simulink model "Model2D"  (R2024b)
settings: Solver=VariableStepAuto  StartTime=0.0  StopTime=10.0  RelTol=1e-3
undefined symbols (not defined in the file or in its folder): AC, Aero, mot, prop, rad, s, Vbi
libraries: aerolibasang x3, aerolibconvert2 x3, aerolibactuator x3, aerolibtransform2 x2, shared6dof x1, aerolibadyn x1, vrlib x1
settings Model: Creator=Tyler  LastModifiedBy=Tyler

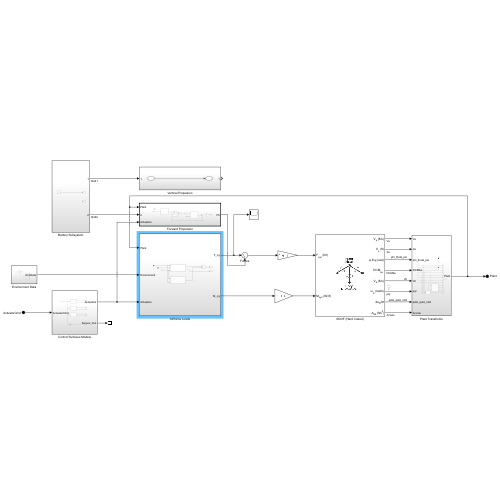
[thumbnail: Simulink's stored preview of the top-level diagram]
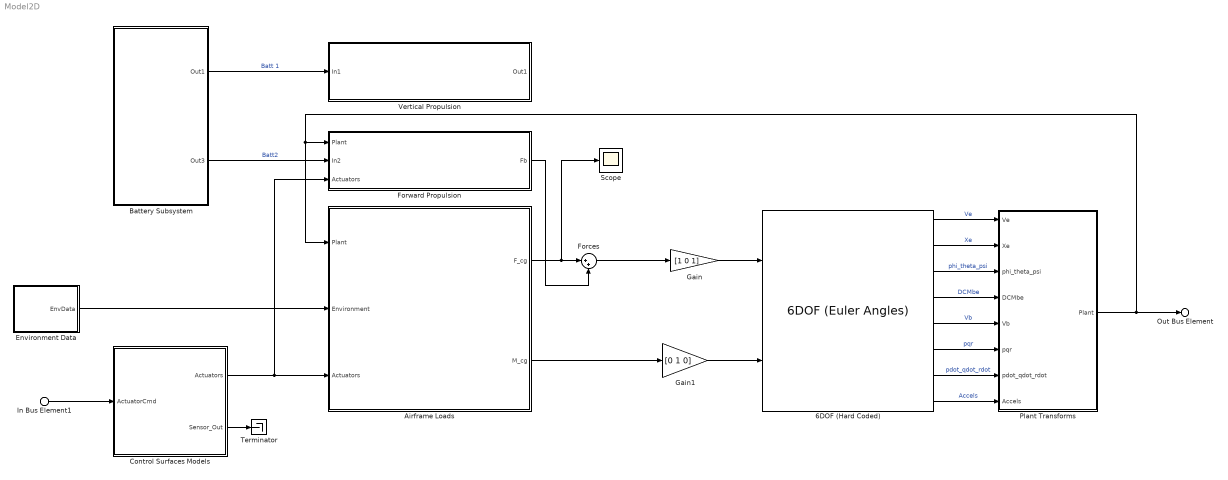
== system Model2D ==
  In Bus Element1 : Inport  PortName=ActuatorCmd
  6DOF (Hard Coded) : shared6dof/6DOF (Euler Angles)  units=English (Velocity in ft/s)  mtype=Fixed  rep=Quaternion  xme_0=[0 0 0]  Vm_0=[0 0 0]  eul_0=[0 0 0]  pm_0=[0 0 0]  mass_0=0.115  mass_e=0.5  mass_f=2.0  inertia=diag([11.38 9.6 20.40])  inertia_e=eye(3)  inertia_f=2*eye(3)  k_quat=1.0  vre_flag=on  abi_flag=off  aMode=0  xme_statename=''  Vm_statename=''  eul_statename=''  quat_statename=''  pm_statename=''  mass_statename=''
  Airframe Loads : Subsystem
  Battery Subsystem : Subsystem
  Control Surfaces Models : Subsystem
  Environment Data : Subsystem
  Forces : Sum  Inputs=|++
  Forward Propulsion : Subsystem  TreatAsAtomicUnit=on
  Gain : Gain  Gain=[1 0 1]
  Gain1 : Gain  Gain=[0 1 0]
  Plant Transforms : Subsystem
  Scope : Scope
  Terminator : Terminator
  Vertical Propulsion : Subsystem
  Out Bus Element : Outport  PortName=Plant
  wires:
  Control Surfaces Models/1(Actuators) -> Airframe Loads/3(Actuators), Forward Propulsion/3(Actuators)
  6DOF (Hard Coded)/6 -> Plant Transforms/6(pqr)  "pqr"
  6DOF (Hard Coded)/3 -> Plant Transforms/3(phi_theta_psi)  "phi_theta_psi"
  6DOF (Hard Coded)/1 -> Plant Transforms/1(Ve)  "Ve"
  Battery Subsystem/2(Out3) -> Forward Propulsion/2(In2)  "Batt2"
  Plant Transforms/1(Plant) -> Out Bus Element/1, Airframe Loads/1(Plant), Forward Propulsion/1(Plant)
  Forward Propulsion/1(Fb) -> Forces/2
  6DOF (Hard Coded)/8 -> Plant Transforms/8(Accels)  "Accels"
  6DOF (Hard Coded)/7 -> Plant Transforms/7(pdot_qdot_rdot)  "pdot_qdot_rdot"
  Gain/1 -> 6DOF (Hard Coded)/1
  6DOF (Hard Coded)/5 -> Plant Transforms/5(Vb)  "Vb"
  Forces/1 -> Gain/1
  Environment Data/1(EnvData) -> Airframe Loads/2(Environment)
  Gain1/1 -> 6DOF (Hard Coded)/2
  6DOF (Hard Coded)/4 -> Plant Transforms/4(DCMbe)  "DCMbe"
  Airframe Loads/2(M_cg) -> Gain1/1
  Control Surfaces Models/2(Sensor_Out) -> Terminator/1
  6DOF (Hard Coded)/2 -> Plant Transforms/2(Xe)  "Xe"
  In Bus Element1/1 -> Control Surfaces Models/1(ActuatorCmd)
  Battery Subsystem/1(Out1) -> Vertical Propulsion/1(In1)  "Batt 1"
  Airframe Loads/1(F_cg) -> Scope/1, Forces/1

== system Model2D/Airframe Loads ==
  Plant : Inport
  In Bus Element : Inport  Port=2  PortName=Environment
  In Bus Element1 : Inport  Port=3  PortName=Actuators
  Add : Sum
  Aerodynamic Loads : Subsystem
  Gravity Force : Subsystem
  F_cg : Outport
  M_cg : Outport  Port=2
  wires:
  Plant/1 -> Gravity Force/1(Plant), Aerodynamic Loads/3(plant)
  In Bus Element/1 -> Gravity Force/2(Environment), Aerodynamic Loads/1(EnvData)
  In Bus Element1/1 -> Aerodynamic Loads/2(Actuators)
  Aerodynamic Loads/1(Fb) -> Add/1
  Add/1 -> F_cg/1
  Aerodynamic Loads/2(Mb) -> M_cg/1
  Gravity Force/1(Fg_b) -> Add/2

== system Model2D/Battery Subsystem ==
  Initial Voltage : Constant
  Out1 : Outport
  Out3 : Outport  Port=2
  wires:
  Initial Voltage/1 -> Out1/1

== system Model2D/Control Surfaces Models ==
  In Bus Element1 : Inport  PortName=ActuatorCmd
  Ailerons : Subsystem
  Bus Selector : BusSelector  OutputSignals=Throttle
  Elevator : Subsystem
  Rudder : Subsystem
  Out Bus Element2 : Outport  VectorParamsAs1DForOutWhenUnconnected=off  PortName=Actuators  Element=Aileron
  Out Bus Element3 : Outport  VectorParamsAs1DForOutWhenUnconnected=off  PortName=Actuators  Element=Elevator
  Out Bus Element4 : Outport  VectorParamsAs1DForOutWhenUnconnected=off  PortName=Actuators  Element=Rudder
  BusElementOut : Outport  PortName=Actuators  Element=Throttle
  Out Bus Element12 : Outport  Port=2  VectorParamsAs1DForOutWhenUnconnected=off  PortName=Sensor_Out  Element=Ail
  Out Bus Element1 : Outport  Port=2  VectorParamsAs1DForOutWhenUnconnected=off  PortName=Sensor_Out  Element=Ele
  Out Bus Element5 : Outport  Port=2  VectorParamsAs1DForOutWhenUnconnected=off  PortName=Sensor_Out  Element=Rud
  wires:
  Ailerons/1(SensorOut) -> Out Bus Element12/1  "Rudder"
  Ailerons/2(Positions) -> Out Bus Element2/1  "Rudder"
  In Bus Element1/1 -> Bus Selector/1, Rudder/1(Commands), Elevator/1(Commands), Ailerons/1(Commands)
  Elevator/1(SensorOut) -> Out Bus Element1/1  "Rudder"
  Elevator/2(Positions) -> Out Bus Element3/1  "Rudder"
  Rudder/2(Positions) -> Out Bus Element4/1  "Rudder"
  Rudder/1(SensorOut) -> Out Bus Element5/1  "Rudder"
  Bus Selector/1 -> BusElementOut/1  "<Throttle>"

== system Model2D/Environment Data ==
  Air Density : Constant  Value=0.002377
  Bus Creator : BusCreator  Inputs=5
  Constant : Constant  Value=0
  Constant1 : Constant  Value=0
  Constant2 : Constant  Value=32.2
  Gravity Acceleration : Constant  Value=[0 0 32.2]
  Mux : Mux  Inputs=3
  Speed of Sound : Constant  Value=1100
  Wind Angular Rates : Constant  Value=[0 0 0]
  Wind Velocity : Constant  Value=[0 0 0]
  EnvData : Outport
  wires:
  Air Density/1 -> Bus Creator/3  "rho"
  Speed of Sound/1 -> Bus Creator/2  "a"
  Mux/1 -> Bus Creator/1  "Ag"
  Wind Velocity/1 -> Bus Creator/4  "WindVelocity"
  Wind Angular Rates/1 -> Bus Creator/5  "WindAngularRates"
  Bus Creator/1 -> EnvData/1  "Environment"
  Constant/1 -> Mux/1
  Constant1/1 -> Mux/2
  Constant2/1 -> Mux/3

== system Model2D/Forward Propulsion ==
  In Bus Element2 : Inport  PortName=Plant  Element=Airspeed
  In2 : Inport  Port=2
  In Bus Element1 : Inport  Port=3  PortName=Actuators  Element=Throttle
  Bus Selector1 : BusSelector  OutputSignals=Thrust,Torque
  Divide1 : Product  Inputs=*/
  Gain1 : Gain  Gain=[1 0 0]
  Integrator : Integrator  InitialCondition=200
  Motor Model : Subsystem
  Prop MOI (slug-ft^2) : Constant  Value=prop.MOI
  Propeller Model : Subsystem
  Subtract : Sum  Inputs=+-
  Fb : Outport
  wires:
  In Bus Element2/1 -> Propeller Model/2(Airspeed)
  Propeller Model/1(Propulsion Data) -> Bus Selector1/1
  Prop MOI (slug-ft^2)/1 -> Divide1/2
  Divide1/1 -> Integrator/1  "Omega dot"
  In Bus Element1/1 -> Motor Model/1(Throttle)
  Integrator/1 -> Propeller Model/1(Omega)  "omega"
  Subtract/1 -> Divide1/1
  Motor Model/1(Torque (ft-lbf)) -> Subtract/1
  Bus Selector1/2 -> Subtract/2  "<Torque>"
  Bus Selector1/1 -> Gain1/1  "<Thrust>"
  Gain1/1 -> Fb/1

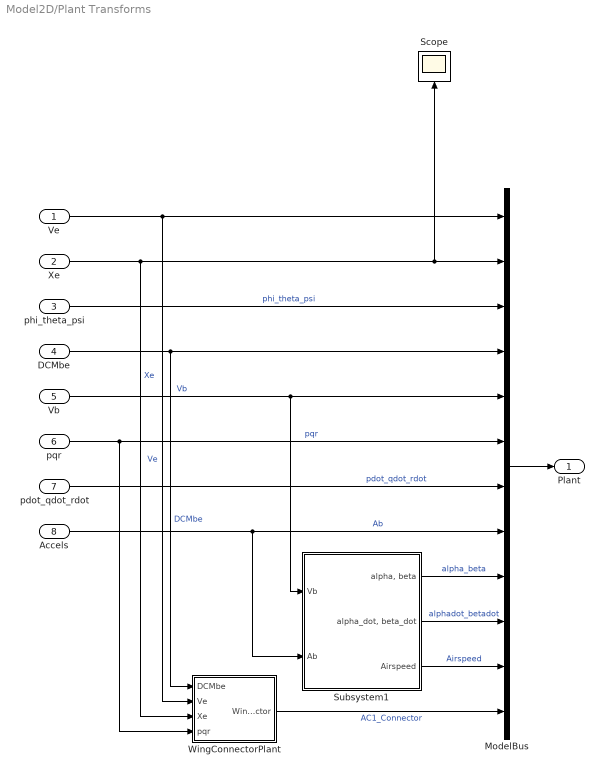
== system Model2D/Plant Transforms ==
  Ve : Inport
  Xe : Inport  Port=2
  phi_theta_psi : Inport  Port=3
  DCMbe : Inport  Port=4
  Vb : Inport  Port=5
  pqr : Inport  Port=6
  pdot_qdot_rdot : Inport  Port=7
  Accels : Inport  Port=8
  ModelBus : BusCreator  Inputs=12
  Scope : Scope
  Subsystem1 : Subsystem
  WingConnectorPlant : Subsystem
  Plant : Outport
  wires:
  Ve/1 -> WingConnectorPlant/2(Ve), ModelBus/1  "Ve"
  ModelBus/1 -> Plant/1
  DCMbe/1 -> ModelBus/4, WingConnectorPlant/1(DCMbe)  "DCMbe"
  pqr/1 -> WingConnectorPlant/4(pqr), ModelBus/6  "pqr"
  pdot_qdot_rdot/1 -> ModelBus/7  "pdot_qdot_rdot"
  Subsystem1/2("alpha_dot, beta_dot") -> ModelBus/10  "alphadot_betadot"
  WingConnectorPlant/1(WingConnector) -> ModelBus/12  "AC1_Connector"
  Xe/1 -> WingConnectorPlant/3(Xe), ModelBus/2, Scope/1  "Xe"
  Subsystem1/1("alpha, beta") -> ModelBus/9  "alpha_beta"
  phi_theta_psi/1 -> ModelBus/3  "phi_theta_psi"
  Accels/1 -> Subsystem1/2(Ab), ModelBus/8  "Ab"
  Vb/1 -> Subsystem1/1(Vb), ModelBus/5  "Vb"
  Subsystem1/3(Airspeed) -> ModelBus/11  "Airspeed"

== system Model2D/Vertical Propulsion ==
  In1 : Inport
  Out1 : Outport
  wires:
  In1/1 -> Out1/1

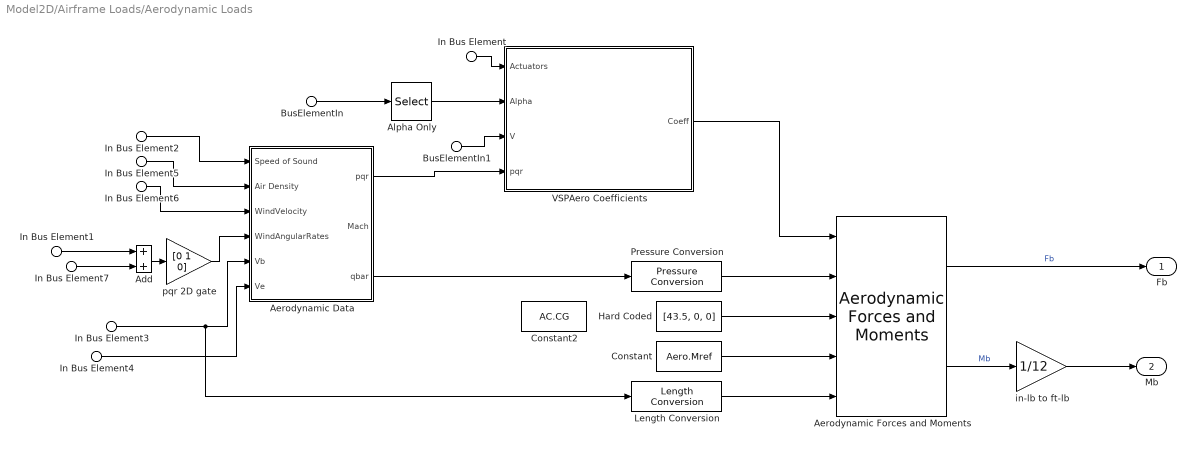
== system Model2D/Airframe Loads/Aerodynamic Loads ==
  In Bus Element6 : Inport  PortName=EnvData  Element=WindVelocity
  In Bus Element7 : Inport  PortName=EnvData  Element=WindAngularRates
  In Bus Element2 : Inport  PortName=EnvData  Element=a
  In Bus Element5 : Inport  PortName=EnvData  Element=rho
  In Bus Element : Inport  Port=2  PortName=Actuators
  In Bus Element3 : Inport  Port=3  PortName=plant  Element=Vb
  In Bus Element4 : Inport  Port=3  PortName=plant  Element=Ve
  In Bus Element1 : Inport  Port=3  PortName=plant  Element=pqr
  BusElementIn : Inport  Port=3  PortName=plant  Element=alpha_beta
  BusElementIn1 : Inport  Port=3  PortName=plant  Element=Airspeed
  Add : Sum
  Aerodynamic Forces and Moments : aerolibadyn/Aerodynamic Forces and Moments   inputAxes=Wind  outputForceAxes=Body  outputMomentAxes=Body  S=Aero.Sref  b=Aero.bref  cbar=Aero.Cref
  Aerodynamic Data : Subsystem
  Alpha Only : Selector  InputPortWidth=2  IndexOptions=Index vector (dialog)  Indices=[1]  OutputSizes=1
  Constant : Constant  Value=Aero.Mref
  Constant2 : Constant  Value=AC.CG
  Hard Coded : Constant  Value=[43.5, 0, 0]
  Length Conversion : aerolibconvert2/Length Conversion  IU=ft  OU=in
  Pressure Conversion : aerolibconvert2/Pressure Conversion  IU=psf  OU=psi
  VSPAero Coefficients : Subsystem
  in-lb to ft-lb : Gain  Gain=1/12
  pqr 2D gate : Gain  Gain=[0 1 0]
  Fb : Outport  VectorParamsAs1DForOutWhenUnconnected=off
  Mb : Outport  Port=2  VectorParamsAs1DForOutWhenUnconnected=off
  wires:
  In Bus Element6/1 -> Aerodynamic Data/3(WindVelocity)
  Aerodynamic Data/1("pqr ") -> VSPAero Coefficients/4(pqr)
  Aerodynamic Forces and Moments/2 -> in-lb to ft-lb/1  "Mb"
  VSPAero Coefficients/1(Coeff) -> Aerodynamic Forces and Moments/1
  In Bus Element7/1 -> Add/2
  Constant/1 -> Aerodynamic Forces and Moments/4
  In Bus Element5/1 -> Aerodynamic Data/2(Air Density)
  In Bus Element2/1 -> Aerodynamic Data/1(Speed of Sound)
  In Bus Element4/1 -> Aerodynamic Data/6(Ve)
  Aerodynamic Forces and Moments/1 -> Fb/1  "Fb"
  In Bus Element1/1 -> Add/1
  In Bus Element/1 -> VSPAero Coefficients/1(Actuators)
  BusElementIn1/1 -> VSPAero Coefficients/3(V)
  In Bus Element3/1 -> Aerodynamic Data/5(Vb), Length Conversion/1
  Aerodynamic Data/3(qbar) -> Pressure Conversion/1
  Hard Coded/1 -> Aerodynamic Forces and Moments/3
  Pressure Conversion/1 -> Aerodynamic Forces and Moments/2
  Length Conversion/1 -> Aerodynamic Forces and Moments/5
  in-lb to ft-lb/1 -> Mb/1
  BusElementIn/1 -> Alpha Only/1
  Alpha Only/1 -> VSPAero Coefficients/2(Alpha)
  pqr 2D gate/1 -> Aerodynamic Data/4(WindAngularRates)
  Add/1 -> pqr 2D gate/1

== system Model2D/Airframe Loads/Gravity Force ==
  Plant : Inport
  Bus Element In2 : Inport  Port=2  PortName=Environment
  Acc to Force : Gain  Gain=AC.mass  OutDataTypeStr=Inherit: Same as input  ParamDataTypeStr=Inherit: Same as input
  Bus Selector : BusSelector  OutputSignals=DCMbe
  Bus Selector1 : BusSelector  OutputSignals=Ag
  Constant : Constant  Value=[0 0 32.2]
  Fg_body : Product  Multiplication=Matrix(*)
  Fg_b : Outport
  wires:
  Bus Selector/1 -> Fg_body/1  "<DCMbe>"
  Acc to Force/1 -> Fg_body/2
  Plant/1 -> Bus Selector/1
  Bus Element In2/1 -> Bus Selector1/1
  Bus Selector1/1 -> ?  "<Ag>"
  Fg_body/1 -> Fg_b/1
  Constant/1 -> Acc to Force/1

== system Model2D/Control Surfaces Models/Ailerons ==
  In Bus Element4 : Inport  PortName=Commands  Element=Aileron
  Nonlinear Second-Order Actuator1 : aerolibactuator/Nonlinear Second-Order Actuator  wn_fin=10  z_fin=1  fin_max=20*pi/180  fin_min=-20*pi/180  fin_maxrate=90*pi/180  fin_act_0=0  fin_act_vel=0
  Scope : Scope  NumInputPorts=2
  SensorOut : Outport  VectorParamsAs1DForOutWhenUnconnected=off
  Positions : Outport  Port=2  VectorParamsAs1DForOutWhenUnconnected=off
  wires:
  Nonlinear Second-Order Actuator1/1 -> Positions/1, Scope/2, SensorOut/1
  In Bus Element4/1 -> Scope/1, Nonlinear Second-Order Actuator1/1  "Ail"

== system Model2D/Control Surfaces Models/Elevator ==
  In Bus Element4 : Inport  PortName=Commands  Element=Elevator
  Nonlinear Second-Order Actuator1 : aerolibactuator/Nonlinear Second-Order Actuator  wn_fin=10  z_fin=1  fin_max=20*pi/180  fin_min=-20*pi/180  fin_maxrate=90*pi/180  fin_act_0=0  fin_act_vel=0
  SensorOut : Outport  VectorParamsAs1DForOutWhenUnconnected=off
  Positions : Outport  Port=2  VectorParamsAs1DForOutWhenUnconnected=off
  wires:
  Nonlinear Second-Order Actuator1/1 -> Positions/1, SensorOut/1
  In Bus Element4/1 -> Nonlinear Second-Order Actuator1/1  "Ele"

== system Model2D/Control Surfaces Models/Rudder ==
  In Bus Element4 : Inport  PortName=Commands  Element=Rudder
  Nonlinear Second-Order Actuator1 : aerolibactuator/Nonlinear Second-Order Actuator  wn_fin=10  z_fin=1  fin_max=20*pi/180  fin_min=-20*pi/180  fin_maxrate=90*pi/180  fin_act_0=0  fin_act_vel=0
  SensorOut : Outport  VectorParamsAs1DForOutWhenUnconnected=off
  Positions : Outport  Port=2  VectorParamsAs1DForOutWhenUnconnected=off
  wires:
  Nonlinear Second-Order Actuator1/1 -> Positions/1, SensorOut/1
  In Bus Element4/1 -> Nonlinear Second-Order Actuator1/1  "Rud"

== system Model2D/Forward Propulsion/Motor Model ==
  Throttle : Inport
  Divide : Product  Inputs=*/
  Kv (RPM/V) : Constant  Value=mot.Kv
  Max Current : Gain  Gain=mot.amp
  Mot Efficiency : Gain
  Motor Conversion Constant : Gain  Gain=8.3
  SI Conversion : Gain  Gain=.7376
  Torque (ft-lbf) : Outport
  wires:
  Mot Efficiency/1 -> Torque (ft-lbf)/1  "Torque (ft-lbf)"
  Throttle/1 -> Max Current/1
  Kv (RPM/V)/1 -> Divide/2
  Divide/1 -> Motor Conversion Constant/1
  Max Current/1 -> Divide/1
  Motor Conversion Constant/1 -> SI Conversion/1  "Torque (N.m)"
  SI Conversion/1 -> Mot Efficiency/1  "Torque (ft-lbf)"

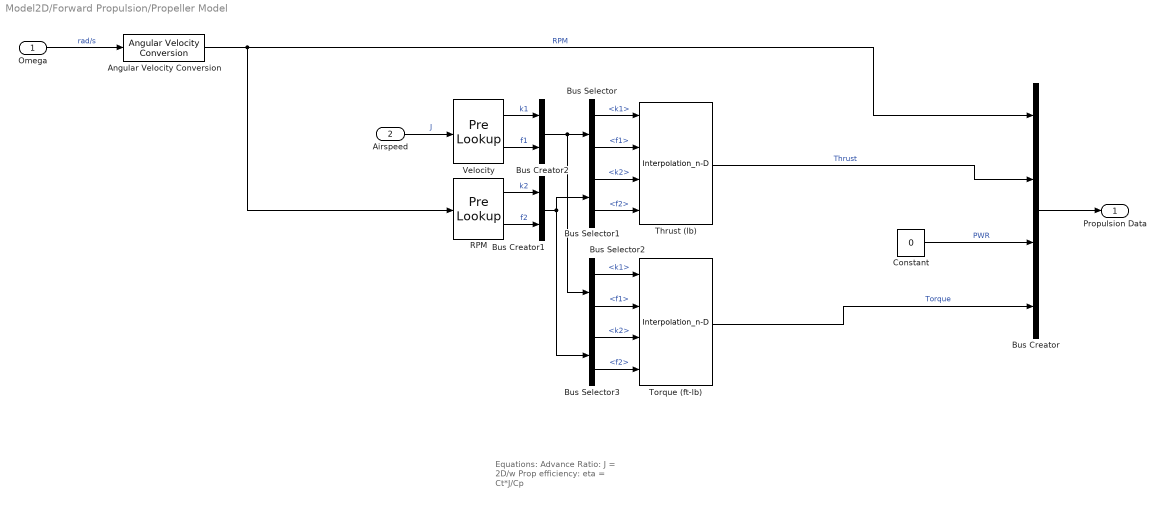
== system Model2D/Forward Propulsion/Propeller Model ==
  note: Equations:
      |
      | Advance Ratio: J = 2D/w
      | Prop efficiency: eta = Ct*J/Cp
  Omega : Inport
  Airspeed : Inport  Port=2
  Angular Velocity Conversion : aerolibconvert2/Angular Velocity Conversion  IU=rad/s  OU=rpm
  Bus Creator : BusCreator  Inputs=4
  Bus Creator1 : BusCreator  Inputs=2
  Bus Creator2 : BusCreator  Inputs=2
  Bus Selector : BusSelector  OutputSignals=k1,f1
  Bus Selector1 : BusSelector  OutputSignals=k2,f2
  Bus Selector2 : BusSelector  OutputSignals=k1,f1
  Bus Selector3 : BusSelector  OutputSignals=k2,f2
  Constant : Constant  Value=0
  RPM : PreLookup  BreakpointsData=prop.RPM  ExtrapMethod=Linear
  Thrust (lb) : Interpolation_n-D  Table=prop.Thrust  InternalRulePriority=Speed
  Torque (ft-lb) : Interpolation_n-D  Table=prop.Torque  ExtrapMethod=Clip  InternalRulePriority=Speed
  Velocity : PreLookup  BreakpointsData=prop.vel
  Propulsion Data : Outport
  wires:
  Constant/1 -> Bus Creator/3  "PWR"
  Torque (ft-lb)/1 -> Bus Creator/4  "Torque"
  Angular Velocity Conversion/1 -> RPM/1, Bus Creator/1  "RPM"
  Bus Creator/1 -> Propulsion Data/1
  Omega/1 -> Angular Velocity Conversion/1  "rad/s"
  Airspeed/1 -> Velocity/1  "J"
  Velocity/2 -> Bus Creator2/2  "f1"
  Bus Creator2/1 -> Bus Selector/1, Bus Selector2/1
  Bus Creator1/1 -> Bus Selector1/1, Bus Selector3/1
  Velocity/1 -> Bus Creator2/1  "k1"
  Bus Selector2/2 -> Torque (ft-lb)/2  "<f1>"
  RPM/1 -> Bus Creator1/1  "k2"
  Bus Selector2/1 -> Torque (ft-lb)/1  "<k1>"
  RPM/2 -> Bus Creator1/2  "f2"
  Thrust (lb)/1 -> Bus Creator/2  "Thrust"
  Bus Selector/2 -> Thrust (lb)/2  "<f1>"
  Bus Selector3/2 -> Torque (ft-lb)/4  "<f2>"
  Bus Selector/1 -> Thrust (lb)/1  "<k1>"
  Bus Selector1/2 -> Thrust (lb)/4  "<f2>"
  Bus Selector3/1 -> Torque (ft-lb)/3  "<k2>"
  Bus Selector1/1 -> Thrust (lb)/3  "<k2>"

== system Model2D/Plant Transforms/Subsystem1 ==
  Vb : Inport
  Ab : Inport  Port=2
  Direction Cosine Matrix Body to Wind : aerolibtransform2/Direction Cosine Matrix Body to Wind
  "Incidence, Sideslip, & Airspeed" : aerolibasang/Incidence, Sideslip, & Airspeed
  Memory4 : Memory  InitialCondition=Vbi
  Mux4 : Mux  Inputs=2
  Product1 : Product  Multiplication=Matrix(*)  InputSameDT=on  SaturateOnIntegerOverflow=on  OutDataTypeStr=Inherit: Same as first input
  "calc alpha_dot, beta_dot" : Subsystem
  "alpha, beta" : Outport  Unit=rad  VectorParamsAs1DForOutWhenUnconnected=off
  "alpha_dot, beta_dot" : Outport  Port=2  Unit=rad/s  VectorParamsAs1DForOutWhenUnconnected=off
  Airspeed : Outport  Port=3
  wires:
  "Incidence, Sideslip, & Airspeed"/2 -> Mux4/2
  Mux4/1 -> "alpha, beta"/1, Direction Cosine Matrix Body to Wind/1, "calc alpha_dot, beta_dot"/1(alpha,beta)
  Direction Cosine Matrix Body to Wind/1 -> Product1/1
  "Incidence, Sideslip, & Airspeed"/1 -> Mux4/1
  Memory4/1 -> Product1/2, "Incidence, Sideslip, & Airspeed"/1
  Product1/1 -> "calc alpha_dot, beta_dot"/3(Vw)
  Ab/1 -> "calc alpha_dot, beta_dot"/2(Ab)
  "Incidence, Sideslip, & Airspeed"/3 -> Airspeed/1
  "calc alpha_dot, beta_dot"/1("alpha_dot, beta_dot") -> "alpha_dot, beta_dot"/1
  Vb/1 -> Memory4/1

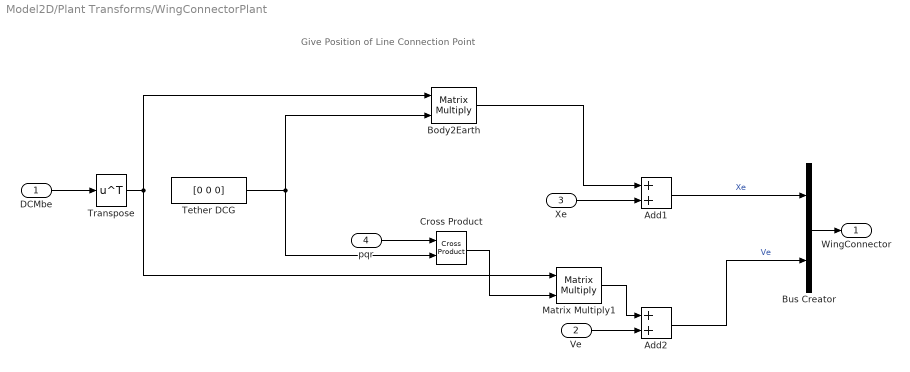
== system Model2D/Plant Transforms/WingConnectorPlant ==
  note: Give Position of Line Connection Point
  DCMbe : Inport
  Ve : Inport  Port=2
  Xe : Inport  Port=3
  pqr : Inport  Port=4
  Add1 : Sum
  Add2 : Sum
  Body2Earth : Product  Multiplication=Matrix(*)
  Bus Creator : BusCreator  Inputs=2
  Cross Product : vrlib/Utilities/Cross Product
  Matrix Multiply1 : Product  Multiplication=Matrix(*)
  Tether DCG : Constant  Value=[0 0 0]
  Transpose : Math  Operator=transpose
  WingConnector : Outport
  wires:
  Bus Creator/1 -> WingConnector/1
  Transpose/1 -> Body2Earth/1, Matrix Multiply1/1
  Body2Earth/1 -> Add1/1
  Add2/1 -> Bus Creator/2  "Ve"
  Xe/1 -> Add1/2
  Matrix Multiply1/1 -> Add2/1
  Tether DCG/1 -> Cross Product/2, Body2Earth/2
  pqr/1 -> Cross Product/1
  Cross Product/1 -> Matrix Multiply1/2
  Add1/1 -> Bus Creator/1  "Xe"
  DCMbe/1 -> Transpose/1
  Ve/1 -> Add2/2

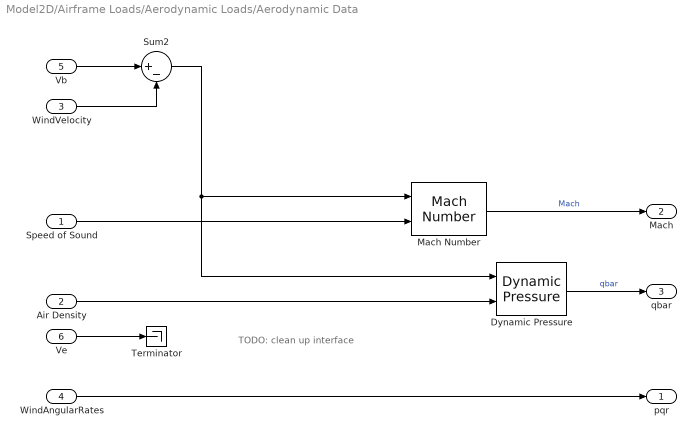
== system Model2D/Airframe Loads/Aerodynamic Loads/Aerodynamic Data ==
  note: TODO: clean up interface
  Speed of Sound : Inport
  Air Density : Inport  Port=2
  WindVelocity : Inport  Port=3  PortDimensions=3
  WindAngularRates : Inport  Port=4  PortDimensions=3
  Vb : Inport  Port=5  PortDimensions=3
  Ve : Inport  Port=6  PortDimensions=3
  Dynamic Pressure : aerolibasang/Dynamic Pressure
  Mach Number : aerolibasang/Mach Number
  Sum2 : Sum  Inputs=|+-  InputSameDT=on  SaturateOnIntegerOverflow=on  OutDataTypeStr=Inherit: Same as first input
  Terminator : Terminator
  "pqr " : Outport  VectorParamsAs1DForOutWhenUnconnected=off
  Mach : Outport  Port=2  VectorParamsAs1DForOutWhenUnconnected=off
  qbar : Outport  Port=3  VectorParamsAs1DForOutWhenUnconnected=off
  wires:
  Dynamic Pressure/1 -> qbar/1  "qbar"
  Sum2/1 -> Mach Number/1, Dynamic Pressure/1
  Ve/1 -> Terminator/1
  Mach Number/1 -> Mach/1  "Mach"
  WindVelocity/1 -> Sum2/2
  Air Density/1 -> Dynamic Pressure/2
  WindAngularRates/1 -> "pqr "/1
  Speed of Sound/1 -> Mach Number/2
  Vb/1 -> Sum2/1

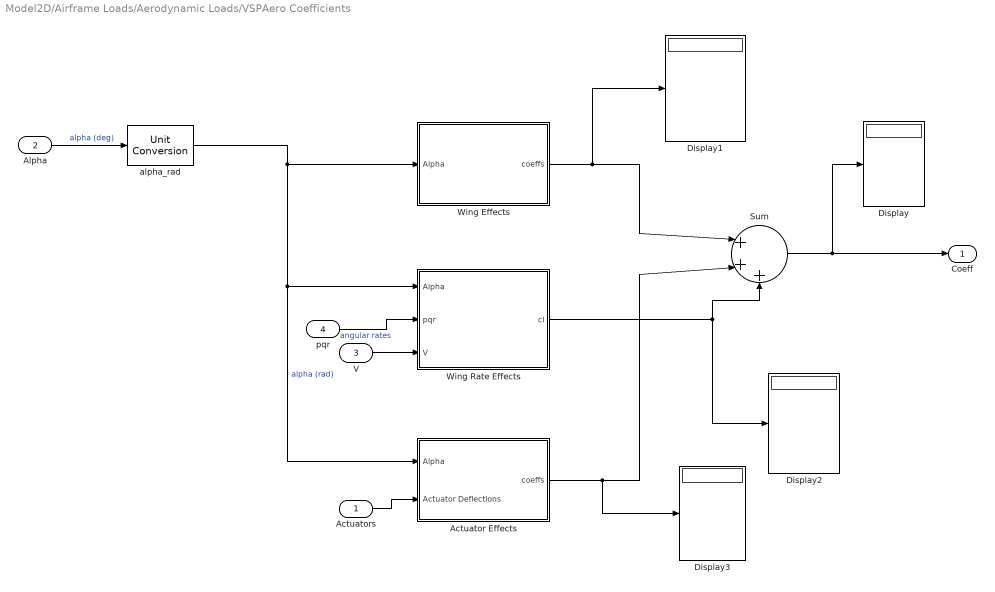
== system Model2D/Airframe Loads/Aerodynamic Loads/VSPAero Coefficients ==
  Actuators : Inport
  Alpha : Inport  Port=2  Unit=rad
  V : Inport  Port=3
  pqr : Inport  Port=4
  Actuator Effects : Subsystem
  Display{,1..3} (4 alike) : Display
  Sum : Sum  Inputs=|+++
  Wing Effects : Subsystem
  Wing Rate Effects : Subsystem
  alpha_rad : UnitConversion
  Coeff : Outport  VectorParamsAs1DForOutWhenUnconnected=off
  wires:
  Wing Rate Effects/1(cl) -> Sum/3, Display2/1
  Sum/1 -> Display/1, Coeff/1
  alpha_rad/1 -> Wing Rate Effects/1(Alpha), Actuator Effects/1(Alpha), Wing Effects/1(Alpha)  "alpha (rad)"
  Actuators/1 -> Actuator Effects/2("Actuator Deflections ")
  V/1 -> Wing Rate Effects/3(V)
  Alpha/1 -> alpha_rad/1  "alpha (deg)"
  Actuator Effects/1(coeffs) -> Sum/2, Display3/1
  pqr/1 -> Wing Rate Effects/2(pqr)  "angular rates"
  Wing Effects/1(coeffs) -> Sum/1, Display1/1

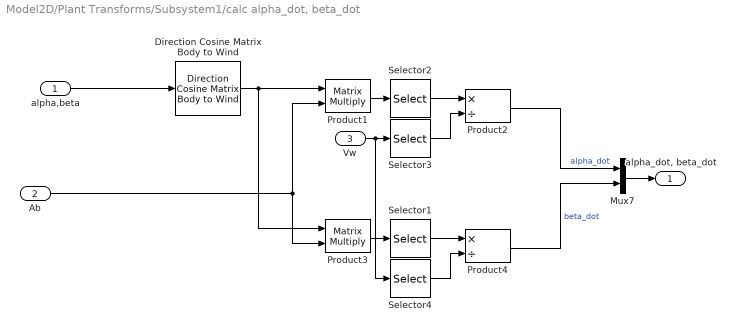
== system Model2D/Plant Transforms/Subsystem1/calc alpha_dot, beta_dot ==
  alpha,beta : Inport
  Ab : Inport  Port=2
  Vw : Inport  Port=3
  Direction Cosine Matrix Body to Wind : aerolibtransform2/Direction Cosine Matrix Body to Wind
  Mux7 : Mux  Inputs=2
  Product1 : Product  Multiplication=Matrix(*)  InputSameDT=on  SaturateOnIntegerOverflow=on  OutDataTypeStr=Inherit: Same as first input
  Product2 : Product  Inputs=*/  InputSameDT=on  SaturateOnIntegerOverflow=on  OutDataTypeStr=Inherit: Same as first input
  Product3 : Product  Multiplication=Matrix(*)  InputSameDT=on  SaturateOnIntegerOverflow=on  OutDataTypeStr=Inherit: Same as first input
  Product4 : Product  Inputs=*/  InputSameDT=on  SaturateOnIntegerOverflow=on  OutDataTypeStr=Inherit: Same as first input
  Selector1 : Selector  IndexMode=Zero-based  InputPortWidth=3  IndexOptions=Index vector (dialog)  Indices=1  OutputSizes=1
  Selector2 : Selector  IndexMode=Zero-based  InputPortWidth=3  IndexOptions=Index vector (dialog)  Indices=2  OutputSizes=1
  Selector3 : Selector  IndexMode=Zero-based  InputPortWidth=3  IndexOptions=Index vector (dialog)  Indices=0  OutputSizes=1
  Selector4 : Selector  IndexMode=Zero-based  InputPortWidth=3  IndexOptions=Index vector (dialog)  Indices=0  OutputSizes=1
  "alpha_dot, beta_dot" : Outport  VectorParamsAs1DForOutWhenUnconnected=off
  wires:
  Product1/1 -> Selector2/1
  Selector2/1 -> Product2/1
  Selector3/1 -> Product2/2
  alpha,beta/1 -> Direction Cosine Matrix Body to Wind/1
  Product2/1 -> Mux7/1  "alpha_dot"
  Ab/1 -> Product1/2, Product3/2
  Vw/1 -> Selector4/1, Selector3/1
  Product4/1 -> Mux7/2  "beta_dot"
  Direction Cosine Matrix Body to Wind/1 -> Product3/1, Product1/1
  Selector1/1 -> Product4/1
  Selector4/1 -> Product4/2
  Product3/1 -> Selector1/1
  Mux7/1 -> "alpha_dot, beta_dot"/1

== system Model2D/Airframe Loads/Aerodynamic Loads/VSPAero Coefficients/Actuator Effects ==
  note: Constant blocks commented out for inputs of finalized model
  Alpha : Inport  Unit=deg
  "Actuator Deflections " : Inport  Port=2
  Add : Sum
  Ailerons : Subsystem
  AlphaLookup : PreLookup  Commented=on  BreakpointsData=Aero.alpha_vec  BeginIndexSearchUsingPreviousIndexResult=on  ExtrapMethod=Linear
  Bus Creator : BusCreator  Commented=on  Inputs=2
  Constant1 : Constant  Commented=on  Value=-30
  Constant3 : Constant  Commented=on  Value=-15
  Display : Display
  Elevator : Subsystem
  coeffs : Outport  VectorParamsAs1DForOutWhenUnconnected=off
  wires:
  Add/1 -> Display/1, coeffs/1
  Ailerons/1(delCoeff) -> Add/2
  AlphaLookup/2 -> Bus Creator/2  "f"
  AlphaLookup/1 -> Bus Creator/1  "k"
  "Actuator Deflections "/1 -> Ailerons/2(Actuators), Elevator/2(Actuators)
  Elevator/1(delCoeff) -> Add/1
  Alpha/1 -> Ailerons/1(Alpha), Elevator/1(Alpha)

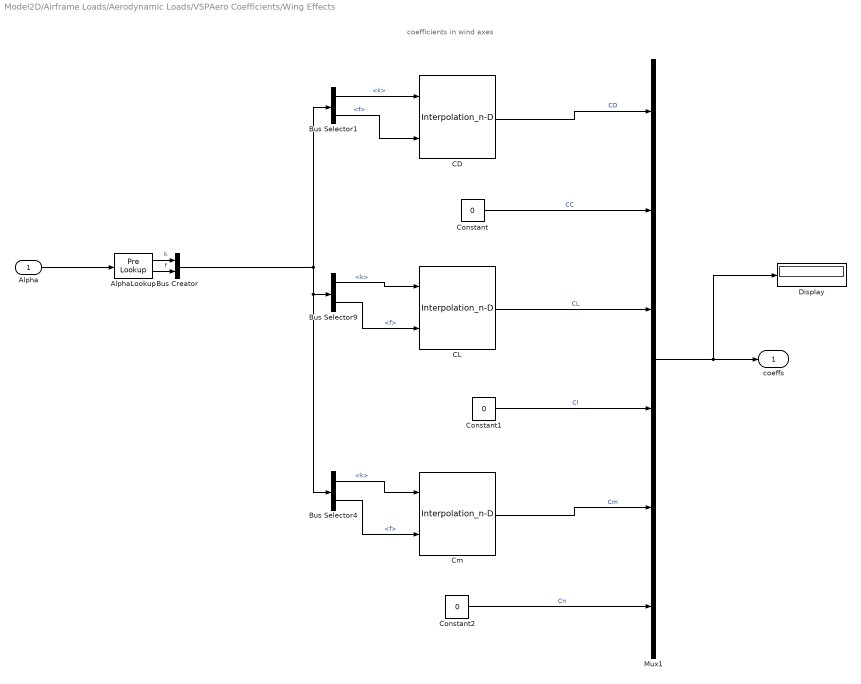
== system Model2D/Airframe Loads/Aerodynamic Loads/VSPAero Coefficients/Wing Effects ==
  note: coefficients in wind axes
  Alpha : Inport  Unit=deg
  AlphaLookup : PreLookup  BreakpointsData=Aero.alpha_vec  BeginIndexSearchUsingPreviousIndexResult=on  ExtrapMethod=Linear
  Bus Creator : BusCreator  Inputs=2
  Bus Selector1 : BusSelector  OutputSignals=k,f
  Bus Selector4 : BusSelector  OutputSignals=k,f
  Bus Selector9 : BusSelector  OutputSignals=k,f
  CD : Interpolation_n-D  NumberOfTableDimensions=1  Table=Aero.CD(find(abs(Aero.beta_vec)==min(abs(Aero.beta_vec)),1),:)  RemoveProtectionIndex=on  SaturateOnIntegerOverflow=on
      settings: InputPortMap=u0,u1
  CL : Interpolation_n-D  NumberOfTableDimensions=1  Table=Aero.CL(find(abs(Aero.beta_vec)==min(abs(Aero.beta_vec)),1),:)  RemoveProtectionIndex=on  SaturateOnIntegerOverflow=on
      settings: InputPortMap=u0,u1
  Cm : Interpolation_n-D  NumberOfTableDimensions=1  Table=Aero.Cm(find(abs(Aero.beta_vec)==min(abs(Aero.beta_vec)),1),:)  RemoveProtectionIndex=on  SaturateOnIntegerOverflow=on
      settings: InputPortMap=u0,u1
  Constant : Constant  Value=0
  Constant1 : Constant  Value=0
  Constant2 : Constant  Value=0
  Display : Display
  Mux1 : Mux  Inputs=6
  coeffs : Outport  VectorParamsAs1DForOutWhenUnconnected=off
  wires:
  AlphaLookup/2 -> Bus Creator/2  "f"
  AlphaLookup/1 -> Bus Creator/1  "k"
  Mux1/1 -> Display/1, coeffs/1
  Alpha/1 -> AlphaLookup/1
  Cm/1 -> Mux1/5  "Cm"
  Bus Selector4/2 -> Cm/2  "<f>"
  Bus Selector1/1 -> CD/1  "<k>"
  CL/1 -> Mux1/3  "CL"
  Bus Selector9/1 -> CL/1  "<k>"
  Bus Selector1/2 -> CD/2  "<f>"
  Constant2/1 -> Mux1/6  "Cn"
  Bus Selector4/1 -> Cm/1  "<k>"
  Bus Creator/1 -> Bus Selector1/1, Bus Selector4/1, Bus Selector9/1
  Constant/1 -> Mux1/2  "CC"
  Bus Selector9/2 -> CL/2  "<f>"
  Constant1/1 -> Mux1/4  "Cl"
  CD/1 -> Mux1/1  "CD"

== system Model2D/Airframe Loads/Aerodynamic Loads/VSPAero Coefficients/Wing Rate Effects ==
  note: Remove these look-up tables when submodels are finalized
  Alpha : Inport  Unit=deg
  pqr : Inport  Port=2
  V : Inport  Port=3
  Aero Surfaces : Subsystem
  AlphaLookup : PreLookup  Commented=on  BreakpointsData=Aero.alpha_vec  BeginIndexSearchUsingPreviousIndexResult=on  ExtrapMethod=Linear
  Bus Creator : BusCreator  Commented=on  Inputs=2
  Display : Display
  Gain : Gain  Gain=Aero.Cref/2
  Product : Product  Inputs=*/
  Scope : Scope
  q only : Selector  InputPortWidth=3  IndexOptions=Index vector (dialog)  Indices=[2]  OutputSizes=1
  cl : Outport  VectorParamsAs1DForOutWhenUnconnected=off
  wires:
  V/1 -> Aero Surfaces/3(V)
  AlphaLookup/2 -> Bus Creator/2  "f"
  AlphaLookup/1 -> Bus Creator/1  "k"
  Aero Surfaces/1(delCoeff) -> Display/1, cl/1, Scope/1
  Alpha/1 -> Aero Surfaces/1(Alpha)
  pqr/1 -> q only/1
  q only/1 -> Gain/1
  Gain/1 -> Product/1

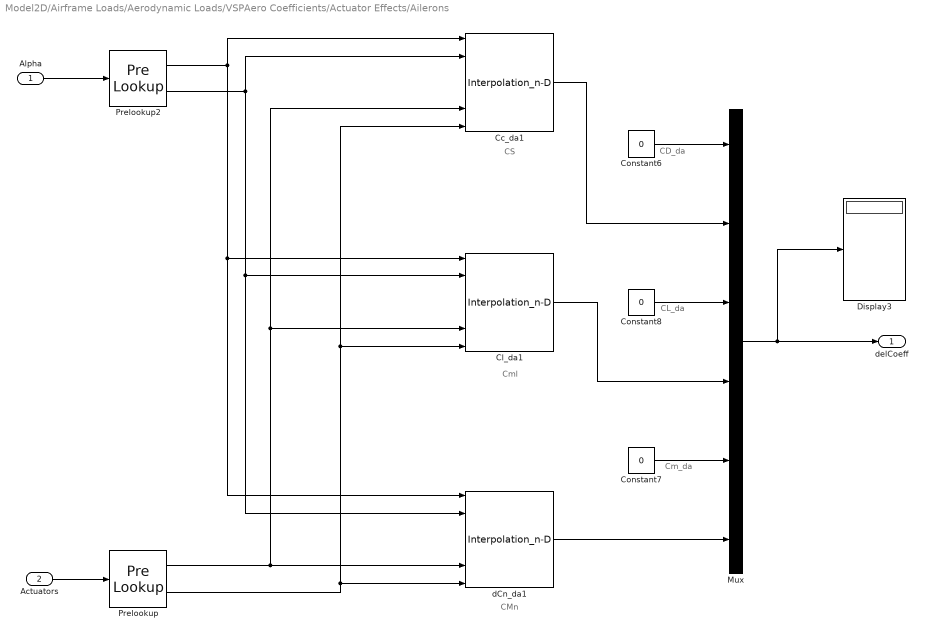
== system Model2D/Airframe Loads/Aerodynamic Loads/VSPAero Coefficients/Actuator Effects/Ailerons ==
  note: CL_da
  note: CD_da
  note: Cm_da
  note: CMn
  note: CS
  note: Cml
  Alpha : Inport
  Actuators : Inport  Port=2
  Cc_da1 : Interpolation_n-D  NumberOfTableDimensions=3  Table=Aero.Cc_da  RemoveProtectionIndex=on  SaturateOnIntegerOverflow=on
      settings: InputPortMap=u0,u1,u2,u3,u4,u5
  Cl_da1 : Interpolation_n-D  NumberOfTableDimensions=3  Table=Aero.Cl_da  RemoveProtectionIndex=on  SaturateOnIntegerOverflow=on
      settings: InputPortMap=u0,u1,u2,u3,u4,u5
  Constant6 : Constant  Value=0
  Constant7 : Constant  Value=0
  Constant8 : Constant  Value=0
  Display3 : Display
  Mux : Mux  Inputs=6
  Prelookup : PreLookup  BreakpointsData=Aero.delta_vec  ExtrapMethod=Linear
  Prelookup2 : PreLookup  BreakpointsData=Aero.alpha_vec  ExtrapMethod=Linear
  dCn_da1 : Interpolation_n-D  NumberOfTableDimensions=3  Table=Aero.Cn_da  RemoveProtectionIndex=on  SaturateOnIntegerOverflow=on
      settings: InputPortMap=u0,u1,u2,u3,u4,u5
  delCoeff : Outport  VectorParamsAs1DForOutWhenUnconnected=off
  wires:
  Constant7/1 -> Mux/5
  Constant6/1 -> Mux/1
  dCn_da1/1 -> Mux/6
  Prelookup2/1 -> dCn_da1/1, Cl_da1/1, Cc_da1/1
  Cc_da1/1 -> Mux/2
  Mux/1 -> delCoeff/1, Display3/1
  Prelookup/1 -> Cc_da1/5, Cl_da1/5, dCn_da1/5
  Prelookup/2 -> Cc_da1/6, Cl_da1/6, dCn_da1/6
  Constant8/1 -> Mux/3
  Prelookup2/2 -> dCn_da1/2, Cl_da1/2, Cc_da1/2
  Cl_da1/1 -> Mux/4
  Actuators/1 -> Prelookup/1
  Alpha/1 -> Prelookup2/1

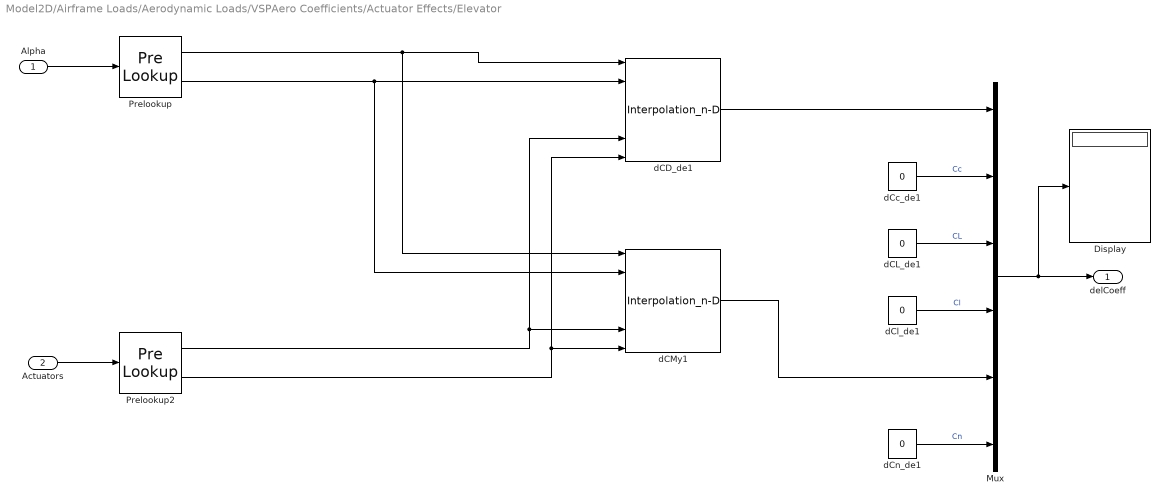
== system Model2D/Airframe Loads/Aerodynamic Loads/VSPAero Coefficients/Actuator Effects/Elevator ==
  Alpha : Inport
  Actuators : Inport  Port=2
  Display : Display
  Mux : Mux  Inputs=6
  Prelookup : PreLookup  BreakpointsData=Aero.alpha_vec  ExtrapMethod=Linear
  Prelookup2 : PreLookup  BreakpointsData=Aero.delta_vec  ExtrapMethod=Linear
  dCD_de1 : Interpolation_n-D  NumberOfTableDimensions=3  Table=Aero.CD_de  RemoveProtectionIndex=on  SaturateOnIntegerOverflow=on
      settings: InputPortMap=u0,u1,u2,u3,u4,u5
  dCL_de1 : Constant  Value=0
  dCMy1 : Interpolation_n-D  NumberOfTableDimensions=3  Table=Aero.Cm_de  RemoveProtectionIndex=on  SaturateOnIntegerOverflow=on
      settings: InputPortMap=u0,u1,u2,u3,u4,u5
  dCc_de1 : Constant  Value=0
  dCl_de1 : Constant  Value=0
  dCn_de1 : Constant  Value=0
  delCoeff : Outport  VectorParamsAs1DForOutWhenUnconnected=off
  wires:
  dCMy1/1 -> Mux/5
  dCn_de1/1 -> Mux/6  "Cn"
  Alpha/1 -> Prelookup/1
  Prelookup2/1 -> dCMy1/5, dCD_de1/5
  Prelookup2/2 -> dCD_de1/6, dCMy1/6
  Prelookup/2 -> dCMy1/2, dCD_de1/2
  dCD_de1/1 -> Mux/1
  dCL_de1/1 -> Mux/3  "CL"
  Prelookup/1 -> dCMy1/1, dCD_de1/1
  dCl_de1/1 -> Mux/4  "Cl"
  Actuators/1 -> Prelookup2/1
  dCc_de1/1 -> Mux/2  "Cc"
  Mux/1 -> delCoeff/1, Display/1

== system Model2D/Airframe Loads/Aerodynamic Loads/VSPAero Coefficients/Wing Rate Effects/Aero Surfaces ==
  note: Display used here to show the Damping Coefficients
      | as a means of ensuring roll, pitch, and yaw rate is correct.
  note: Display for the C_roll, C_pitch, and C_yaw after convert/add.
  Alpha : Inport
  pqr : Inport  Port=2
  V : Inport  Port=3
  Bus Creator : BusCreator  Inputs=3
  "C_roll, C_pitch, C_yaw" : Display
  Coefs Due to Pitch Rate : Subsystem
  Convert & Add : Subsystem
      settings: PortSchema="{\"entries\":[{\"content\":{\"sides\":[{\"content\":{\"connectorIds\":[\"In1\"]},\"type\":\"ConnectorPlacement.EquallySpacedRectSide\",\"uuid\":\"b8013de1-6e73-47c3-a52d-200a37bea422\"},{\"content\":{\"connectorIds\":[\"Out1\"],\"side\":\"RIGHT\"},\"type\":\"ConnectorPlacement.EquallySpacedRectSide\",\"uuid\":\"fcf5ea14-4050-433a-82d6-0b7656ed6099\"},{\"content\":{\"connectorIds\":[\"In2\",\"In3\"],\"side\":\"TOP\"},\"type\":\"ConnectorPlacement.EquallySpacedRectSide\",\"uuid\":\"1c09a769-a85c-46fb-a83d-04bd39ae92ac\"},{\"content\":{\"side\":\"BOTTOM\"},\"type\":\"ConnectorPlacement.EquallySpacedRectSide\",\"uuid\":\"8f4a7c03-2c0e-435b-85d5-b3305cee738f\"}]},\"type\":\"ConnectorPlacement.EquallySpacedConnector\",\"uuid\":\"e7daaf90-0c94-4b5f-ae16-89aa994c358a\"}],\"packageUris\":[\"http://schema.mathworks.com/mf0/Connector/R2020b\"],\"version\":\"1.0\"}"
  Display : Display
  delCoeff : Outport  VectorParamsAs1DForOutWhenUnconnected=off
  wires:
  Bus Creator/1 -> Display/1  "Damp Coef"
  Convert & Add/1(delCoeff) -> "C_roll, C_pitch, C_yaw"/1, delCoeff/1
  Alpha/1 -> Coefs Due to Pitch Rate/1(Alpha)
  V/1 -> Convert & Add/3(V)
  pqr/1 -> Convert & Add/2(pqr)

== system Model2D/Airframe Loads/Aerodynamic Loads/VSPAero Coefficients/Wing Rate Effects/Aero Surfaces/Coefs Due to Pitch Rate ==
  Alpha : Inport
  Cm_q1 : Interpolation_n-D  Table=Aero.Cm_q  ExtrapMethod=Clip  RemoveProtectionIndex=on  SaturateOnIntegerOverflow=on
  Constant{5..9} (5 alike) : Constant  Value=0
  Display : Display
  Gain1 : Gain  Commented=through  Gain=0.1
  Mux2 : Mux  Inputs=6
  Prelookup : PreLookup  BreakpointsData=Aero.alpha_vec  ExtrapMethod=Linear
  Out1 : Outport
  wires:
  Alpha/1 -> Prelookup/1
  Cm_q1/1 -> Gain1/1  "CMy"
  Constant5/1 -> Mux2/2  "Cc_q"
  Constant6/1 -> Mux2/4  "Cl_q"
  Constant7/1 -> Mux2/6  "Cn_q"
  Gain1/1 -> Mux2/5  "Cm_q"
  Mux2/1 -> Out1/1, Display/1
  Prelookup/1 -> Cm_q1/3
  Prelookup/2 -> Cm_q1/4
  Constant8/1 -> Mux2/1  "CD_q"
  Constant9/1 -> Mux2/3  "CL_q"

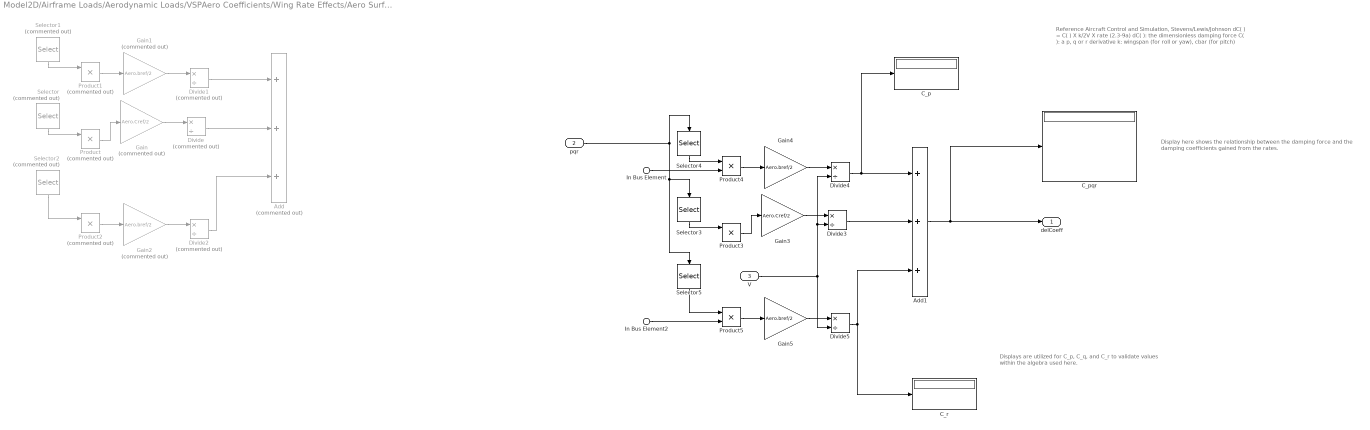
== system Model2D/Airframe Loads/Aerodynamic Loads/VSPAero Coefficients/Wing Rate Effects/Aero Surfaces/Convert & Add ==
  note: Displays are utilized for C_p, C_q, and C_r to validate values
      | within the algebra used here.
  note: Display here shows the relationship between the damping force and
      | the damping coefficients gained from the rates.
  note: Reference Aircraft Control and Simulation, Stevens/Lewis/Johnson
      | dC( ) = C( ) X k/2V X rate    (2.3-9a)
      |
      | dC( ): the dimensionless damping force
      | C( ): a p, q or r derivative
      | k: wingspan (for roll or yaw), cbar (for pitch)
  In Bus Element : Inport  PortName=DampCoef  Element=C()_p
  In Bus Element2 : Inport  PortName=DampCoef  Element=C()_r
  pqr : Inport  Port=2
  V : Inport  Port=3
  Add : Sum  Commented=on  Inputs=+++
  Add1 : Sum  Inputs=+++
  C_p : Display
  C_pqr : Display
  C_r : Display
  Divide : Product  Commented=on  Inputs=*/
  Divide1 : Product  Commented=on  Inputs=*/
  Divide2 : Product  Commented=on  Inputs=*/
  Divide3 : Product  Inputs=*/
  Divide4 : Product  Inputs=*/
  Divide5 : Product  Inputs=*/
  Gain : Gain  Commented=on  Gain=Aero.Cref/2
  Gain1 : Gain  Commented=on  Gain=Aero.bref/2
  Gain2 : Gain  Commented=on  Gain=Aero.bref/2
  Gain3 : Gain  Gain=Aero.Cref/2
  Gain4 : Gain  Gain=Aero.bref/2
  Gain5 : Gain  Gain=Aero.bref/2
  Product : Product  Commented=on
  Product1 : Product  Commented=on
  Product2 : Product  Commented=on
  Product3 : Product
  Product4 : Product
  Product5 : Product
  Selector : Selector  Commented=on  InputPortWidth=3  IndexOptions=Index vector (dialog)  Indices=[ 2]  OutputSizes=1
  Selector1 : Selector  Commented=on  InputPortWidth=3  IndexOptions=Index vector (dialog)  Indices=[ 1]  OutputSizes=1
  Selector2 : Selector  Commented=on  InputPortWidth=3  IndexOptions=Index vector (dialog)  Indices=[ 3]  OutputSizes=1
  Selector3 : Selector  InputPortWidth=3  IndexOptions=Index vector (dialog)  Indices=[ 2]  OutputSizes=1
  Selector4 : Selector  InputPortWidth=3  IndexOptions=Index vector (dialog)  Indices=[ 1]  OutputSizes=1
  Selector5 : Selector  InputPortWidth=3  IndexOptions=Index vector (dialog)  Indices=[ 3]  OutputSizes=1
  delCoeff : Outport
  wires:
  Divide1/1 -> Add/1
  Selector/1 -> Product/1
  Selector1/1 -> Product1/1
  Gain1/1 -> Divide1/1
  Product1/1 -> Gain1/1
  Gain/1 -> Divide/1
  Product/1 -> Gain/1
  Divide/1 -> Add/2
  Divide2/1 -> Add/3
  Gain2/1 -> Divide2/1
  Product2/1 -> Gain2/1
  Selector2/1 -> Product2/1
  In Bus Element2/1 -> Product5/2
  Selector3/1 -> Product3/1
  Gain4/1 -> Divide4/1
  Product4/1 -> Gain4/1
  Gain3/1 -> Divide3/1
  Selector5/1 -> Product5/1
  pqr/1 -> Selector4/1, Selector5/1, Selector3/1
  Divide3/1 -> Add1/2
  Divide5/1 -> Add1/3, C_r/1
  Selector4/1 -> Product4/1
  In Bus Element/1 -> Product4/2
  Product3/1 -> Gain3/1
  Product5/1 -> Gain5/1
  Add1/1 -> delCoeff/1, C_pqr/1
  Gain5/1 -> Divide5/1
  Divide4/1 -> C_p/1, Add1/1
  V/1 -> Divide3/2, Divide4/2, Divide5/2
